simulink model "feedback_harness"  (R2019a)
settings: Solver=FixedStepAuto  StartTime=0.0  StopTime=120  FixedStep=0.001  RelTol=1e-3
settings Model: ModifiedByFormat=The MathWorks Inc.  NumberOfSteps=100  SnapshotBufferSize=3  SnapshotInterval=100  Creator=The MathWorks, Inc.  LastModifiedBy=The MathWorks Inc.
settings DataIOCC: LimitDataPoints=on  SaveFormat=Array  SaveOutput=off  SaveTime=off  ReturnWorkspaceOutputs=off
settings OptimizationCC: ExpressionDepthLimit=2147483647  LifeSpan=1
settings DebuggingCC: UnderspecifiedInitializationDetection=Classic  MergeDetectMultiDrivingBlocksExec=none  SolverPrmCheckMsg=warning  FcnCallInpInsideContextMsg=warning  StateNameClashWarn=warning  SFUnexpectedBacktrackingDiag=warning  SFNoUnconditionalDefaultTransitionDiag=warning  SFExecutionAtInitializationDiag=none  ArithmeticOperatorsInVariantConditions=warning
settings HardwareCC: ProdBitPerPointer=32  ProdBitPerSizeT=32  ProdBitPerPtrDiffT=32  ProdLargestAtomicFloat=None  ProdIntDivRoundTo=Undefined  ProdEndianess=Unspecified  ProdWordSize=32  ProdHWDeviceType=32-bit Generic
settings ModelReferenceCC: PropagateSignalLabelsOutOfModel=off
settings SFSimCC: SimUseLocalCustomCode=off
settings RTWCC: RTWUseLocalCustomCode=off
settings CodeAppCC: StateflowObjectComments=on
settings GRTTargetCC: TargetLangStandard=C89/C90 (ANSI)  GeneratePreprocessorConditionals=Disable all  CombineOutputUpdateFcns=off  GRTInterface=on
settings ConfigComp: CovMetricSettings=dw  CovHtmlReporting=on  CovSaveCumulativeToWorkspaceVar=on  CovSaveSingleToWorkspaceVar=on  CovExternalEMLEnable=off  CovSFcnEnable=off

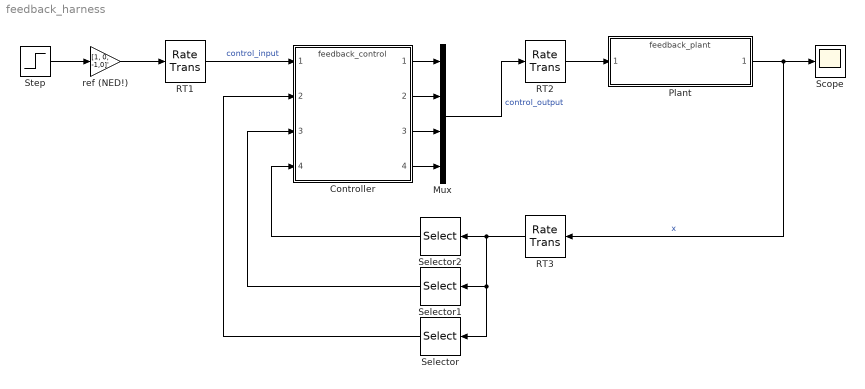
== system feedback_harness ==
  Controller : ModelReference  ModelNameDialog=feedback_control.slx  SimulationMode=Normal  ModelReferenceVersion=1.8
  Mux : Mux
  Plant : ModelReference  ModelNameDialog=feedback_plant.slx  SimulationMode=Normal  ModelReferenceVersion=1.72
  RT1 : RateTransition
  RT2 : RateTransition
  RT3 : RateTransition
  Scope : Scope
  Selector : Selector  InputPortWidth=12  IndexOptions=Index vector (dialog)  Indices=[1:3]  OutputSizes=1
  Selector1 : Selector  InputPortWidth=12  IndexOptions=Index vector (dialog)  Indices=[4:6]  OutputSizes=1
  Selector2 : Selector  InputPortWidth=12  IndexOptions=Index vector (dialog)  Indices=[9:12]  OutputSizes=1
  Step : Step  Time=0  SampleTime=0
  ref (NED!) : Gain  Gain=[1, 0, -1,0]'
  wires:
  Mux/1 -> RT2/1  "control_output"
  Plant/1 -> RT3/1, Scope/1  "x"
  RT1/1 -> Controller/1  "control_input"
  RT2/1 -> Plant/1
  Controller/1 -> Mux/1
  Controller/2 -> Mux/2
  Controller/3 -> Mux/3
  Controller/4 -> Mux/4
  RT3/1 -> Selector2/1, Selector/1, Selector1/1
  Selector2/1 -> Controller/4
  Selector1/1 -> Controller/3
  Selector/1 -> Controller/2
  Step/1 -> ref (NED!)/1
  ref (NED!)/1 -> RT1/1
